simulink model "LMI"  (R2025b)
settings: Solver=VariableStepAuto  StartTime=0.0  StopTime=20.0  RelTol=1e-3
undefined symbols (not defined in the file): A, B, C, D, h0, href, K_LMI, N
settings Model: Creator=salvo  LastModifiedBy=salvo

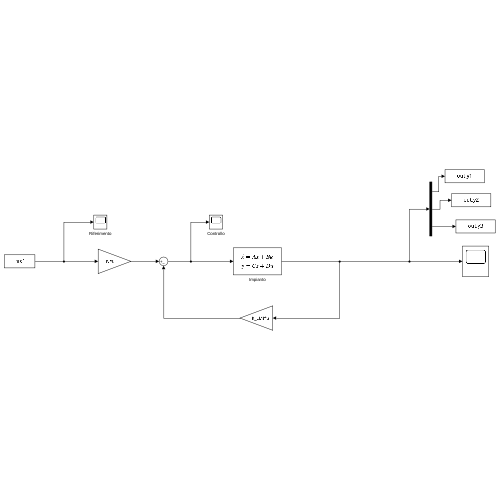
[thumbnail: Simulink's stored preview of the top-level diagram]
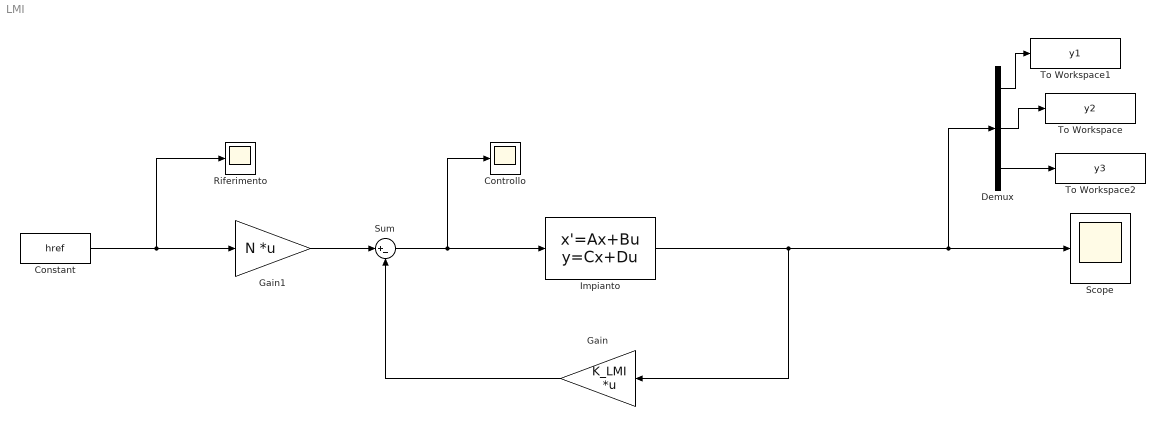
== system LMI ==
  Constant : Constant  Value=href
  Controllo : Scope
      settings: ActiveDisplayYMinimum=-0.20478890790577584  ActiveDisplayYMaximum=-0.01510951782401232  DataLoggingVariableName=ScopeData2
  Demux : Demux  Outputs=3
  Gain : Gain  Gain=K_LMI  Multiplication=Matrix(K*u)
  Gain1 : Gain  Gain=N  Multiplication=Matrix(K*u)
  Impianto : StateSpace  A=A  B=B  C=C  D=D  InitialCondition=h0
  Riferimento : Scope
  Scope : Scope
      settings: ActiveDisplayYMinimum=0.21749037695935816  ActiveDisplayYMaximum=0.26357468477099483
  Sum : Sum  Inputs=|+-
  To Workspace : ToWorkspace  VariableName=y2  SaveFormat=Timeseries  SampleTime=-1
  To Workspace1 : ToWorkspace  VariableName=y1  SaveFormat=Timeseries  SampleTime=-1
  To Workspace2 : ToWorkspace  VariableName=y3  SaveFormat=Timeseries  SampleTime=-1
  wires:
  Sum/1 -> Impianto/1, Controllo/1
  Gain/1 -> Sum/2
  Constant/1 -> Gain1/1, Riferimento/1
  Impianto/1 -> Demux/1, Scope/1, Gain/1
  Demux/1 -> To Workspace1/1
  Demux/2 -> To Workspace/1
  Gain1/1 -> Sum/1
  Demux/3 -> To Workspace2/1
